simulink library "basic_THB"  (Simulink 8.2)
settings: Solver=ode45  StartTime=0.0  StopTime=10.0  RelTol=1e-3
undefined symbols (not defined in the file): dia, fluid, hgt, ID, mdot, mix, p
settings Model: Creator=lena.frank  LastModifiedBy=drhf

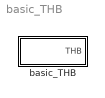
== system basic_THB ==
  basic_THB : Subsystem  mask(constant THV){t=t, mdot=mdot, p=p, ID=ID, fluid=fluid, mix=mix, dia=dia, hgt=hgt}
      mask prompts: t "temperature [degree centigrade]"; mdot "massflow [kg/s]"; p "pressure [Pa]"; ID "Caclulation mode"; mix "fluid mixture [0..1]"; dia "diameter [m]"; hgt "Static height in m"
      mask help:
      | Create a constant Thermo-Hydraulic-Vector.
      | Calculation mode:
      |     1 ..  9999 no pressure drop (dp)
      | 10001 .. 19999 dp caused by flowrate
      | 20001 .. inf   dp by flowrate and static height
      mask init:
      | mix = min(1, max(0, mix));
      | dia = max(dia, 0.001);
      | ID = max(ID,1);
      mask Help: web(fullfile(path_carnot('help'),'basic_THB.html'),'-helpbrowser')

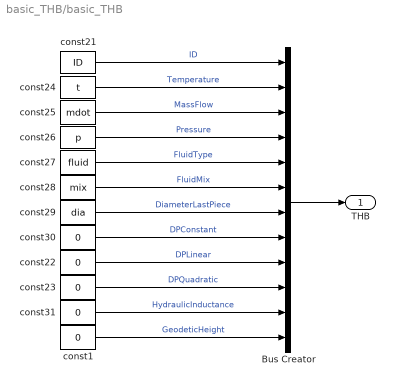
== system basic_THB/basic_THB ==
  Bus Creator : BusCreator  InitFcn=load THB.mat  Inputs=12  OutDataTypeStr=Bus: THB
  const{1,22..23,30..31} (5 alike) : Constant  Value=0
  const21 : Constant  Value=ID
  const24 : Constant  Value=t
  const25 : Constant  Value=mdot
  const26 : Constant  Value=p
  const27 : Constant  Value=fluid
  const28 : Constant  Value=mix
  const29 : Constant  Value=dia
  THB : Outport
  wires:
  const1/1 -> Bus Creator/12  "GeodeticHeight"
  const31/1 -> Bus Creator/11  "HydraulicInductance"
  const23/1 -> Bus Creator/10  "DPQuadratic"
  const22/1 -> Bus Creator/9  "DPLinear"
  Bus Creator/1 -> THB/1
  const21/1 -> Bus Creator/1  "ID"
  const24/1 -> Bus Creator/2  "Temperature"
  const25/1 -> Bus Creator/3  "MassFlow"
  const26/1 -> Bus Creator/4  "Pressure"
  const27/1 -> Bus Creator/5  "FluidType"
  const28/1 -> Bus Creator/6  "FluidMix"
  const29/1 -> Bus Creator/7  "DiameterLastPiece"
  const30/1 -> Bus Creator/8  "DPConstant"
